simulink model "udp_test"  (R2017b)
settings: Solver=FixedStepDiscrete  StartTime=0.0  StopTime=inf  FixedStep=0.005  RelTol=1e-3
InitFcn:
  | PreFunctions.PreParams
libraries: xpcutilitieslib x1, xpcrtudplib x1
settings Model: SimulationMode=external  Creator=hanli  LastModifiedBy=taizun
settings DataIOCC: SaveFormat=StructureWithTime
settings OptimizationCC: BlockReduction=off  OptimizeBlockIOStorage=off  BufferReuse=off  GlobalBufferReuse=off  ExpressionFolding=off  LocalBlockOutputs=off
settings DebuggingCC: InheritedTsInSrcMsg=none
settings HardwareCC: ProdBitPerPointer=32  ProdBitPerSizeT=32  ProdBitPerPtrDiffT=32  ProdLargestAtomicFloat=None  ProdWordSize=32  ProdLongLongMode=on  ProdHWDeviceType=Generic->32-bit x86 compatible
settings RTWCC: SystemTargetFile=slrt.tlc  TemplateMakefile=slrt_default_tmf  Description=Simulink Real-Time  CustomSource=Jp_toe_joint_right_src.c  CodeExecutionProfiling=on  RTWCompilerOptimization=on
settings SimulinkRealTimeCC: SupportVariableSizeSignals=on  RL32LogTETModifier=off  xPCConcurrentTasks=on

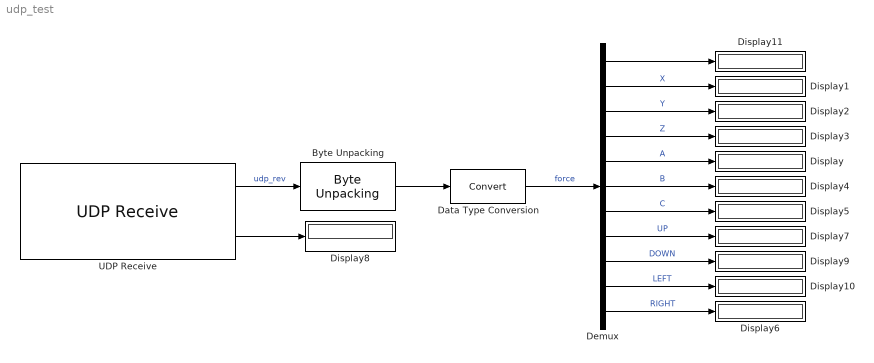
== system udp_test ==
  "Byte Unpacking " : xpcutilitieslib/Byte Unpacking   MaskUnpackedDataTypes={'int8'}  MaskUnpackedDataSizes={[11]}  MaskAlignment=1
      settings: SourceProductName=Simulink Real-Time  SourceProductBaseCode=XP
  Data Type Conversion : DataTypeConversion
  Demux : Demux  Outputs=11
  Display{,1..11} (12 alike) : Display
  UDP Receive : xpcrtudplib/UDP Receive  ipAddressVal=Use host-target connection  localPort=10001  rcvWidth=11  rcvFmAny=on  fmAddress=0.0.0.0  maxUDPQueue=8  sampleTime=0.005
      settings: SourceProductName=Simulink Real-Time
  wires:
  UDP Receive/1 -> "Byte Unpacking "/1  "udp_rev"
  "Byte Unpacking "/1 -> Data Type Conversion/1
  UDP Receive/2 -> Display8/1
  Data Type Conversion/1 -> Demux/1  "force"
  Demux/2 -> Display1/1  "X"
  Demux/3 -> Display2/1  "Y"
  Demux/4 -> Display3/1  "Z"
  Demux/5 -> Display/1  "A"
  Demux/6 -> Display4/1  "B"
  Demux/7 -> Display5/1  "C"
  Demux/8 -> Display7/1  "UP"
  Demux/9 -> Display9/1  "DOWN"
  Demux/10 -> Display10/1  "LEFT"
  Demux/11 -> Display6/1  "RIGHT"
  Demux/1 -> Display11/1
